simulink subsystem "rss_GDVltgHiLvl1Dia"  (R2023a)
settings: Solver=VariableStepAuto  StartTime=0.0  StopTime=10.0  RelTol=1e-3
undefined symbols (not defined in the file): ENM_TYPE_FALT, Gu16_ctGDVltgHiLvl1ConfCnt_C, Gu16_ctGDVltgHiLvl1RcvyCnt_C, Gu16_uGDVltgHiLvl1ConfTrs_C, Gu16_uGDVltgHiLvl1RcvyTrs_C
libraries: vhit_control_library x1, lib_debounce x1, lib_fault_definiteness x1
settings Model: Creator=xiaoqiang.yuan  LastModifiedBy=xiaoqiang.yuan

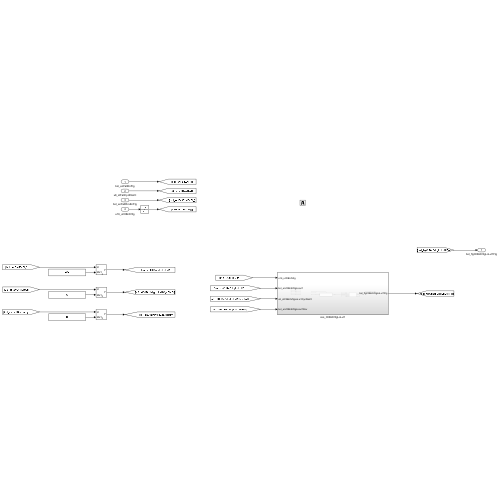
[thumbnail: Simulink's stored preview of the top-level diagram]
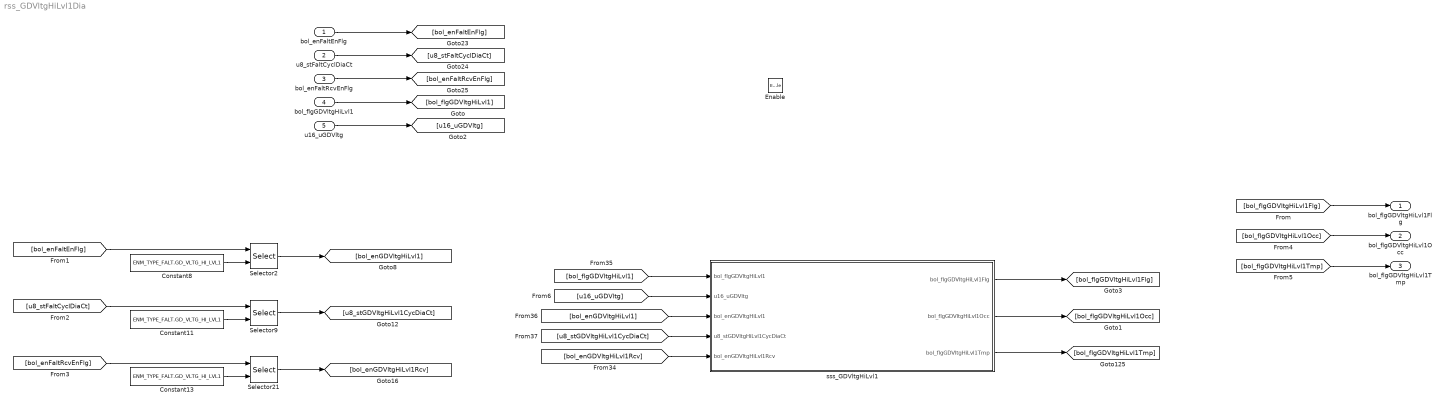
== system rss_GDVltgHiLvl1Dia ==
  bol_enFaltEnFlg : Inport  OutDataTypeStr=boolean
  u8_stFaltCyclDiaCt : Inport  Port=2  OutDataTypeStr=uint8
  bol_enFaltRcvEnFlg : Inport  Port=3  OutDataTypeStr=boolean
  bol_flgGDVltgHiLvl1 : Inport  Port=4  OutDataTypeStr=boolean
  u16_uGDVltg : Inport  Port=5  OutDataTypeStr=dt_Standardize_u16p15b0
  Enable : EnablePort
  Constant11 : Constant  Value=ENM_TYPE_FALT.GD_VLTG_HI_LVL1
  Constant13 : Constant  Value=ENM_TYPE_FALT.GD_VLTG_HI_LVL1
  Constant8 : Constant  Value=ENM_TYPE_FALT.GD_VLTG_HI_LVL1
  Selector2 : Selector  IndexMode=Zero-based  InputPortWidth=Cdbl_numFaltDiaNum  IndexOptions=Index vector (port)  Indices=[1 3]  OutputSizes=1
  Selector21 : Selector  IndexMode=Zero-based  InputPortWidth=Cdbl_numFaltDiaNum  IndexOptions=Index vector (port)  Indices=[1 3]  OutputSizes=1
  Selector9 : Selector  IndexMode=Zero-based  InputPortWidth=Cdbl_numFaltDiaNum  IndexOptions=Index vector (port)  Indices=[1 3]  OutputSizes=1
  sss_GDVltgHiLvl1 : Subsystem
  bol_flgGDVltgHiLvl1Flg : Outport  OutDataTypeStr=boolean
  bol_flgGDVltgHiLvl1Occ : Outport  Port=2  OutDataTypeStr=boolean
  bol_flgGDVltgHiLvl1Tmp : Outport  Port=3  OutDataTypeStr=boolean
  wires:
  [bol_flgGDVltgHiLvl1Flg] -> bol_flgGDVltgHiLvl1Flg/1
  [bol_flgGDVltgHiLvl1] -> sss_GDVltgHiLvl1/1(bol_flgGDVltgHiLvl1)
  [u8_stGDVltgHiLvl1CycDiaCt] -> sss_GDVltgHiLvl1/4(u8_stGDVltgHiLvl1CycDiaCt)
  [bol_enGDVltgHiLvl1] -> sss_GDVltgHiLvl1/3(bol_enGDVltgHiLvl1)
  sss_GDVltgHiLvl1/1(bol_flgGDVltgHiLvl1Flg) -> [bol_flgGDVltgHiLvl1Flg]
  [bol_enGDVltgHiLvl1Rcv] -> sss_GDVltgHiLvl1/5(bol_enGDVltgHiLvl1Rcv)
  u8_stFaltCyclDiaCt/1 -> [u8_stFaltCyclDiaCt]
  bol_enFaltRcvEnFlg/1 -> [bol_enFaltRcvEnFlg]
  bol_enFaltEnFlg/1 -> [bol_enFaltEnFlg]
  [u8_stFaltCyclDiaCt] -> Selector9/1
  [bol_enFaltRcvEnFlg] -> Selector21/1
  [bol_enFaltEnFlg] -> Selector2/1
  Selector21/1 -> [bol_enGDVltgHiLvl1Rcv]
  Selector9/1 -> [u8_stGDVltgHiLvl1CycDiaCt]
  Selector2/1 -> [bol_enGDVltgHiLvl1]
  Constant11/1 -> Selector9/2
  Constant13/1 -> Selector21/2
  Constant8/1 -> Selector2/2
  bol_flgGDVltgHiLvl1/1 -> [bol_flgGDVltgHiLvl1]
  sss_GDVltgHiLvl1/2(bol_flgGDVltgHiLvl1Occ) -> [bol_flgGDVltgHiLvl1Occ]
  [bol_flgGDVltgHiLvl1Occ] -> bol_flgGDVltgHiLvl1Occ/1
  [u16_uGDVltg] -> sss_GDVltgHiLvl1/2(u16_uGDVltg)
  u16_uGDVltg/1 -> [u16_uGDVltg]
  [bol_flgGDVltgHiLvl1Tmp] -> bol_flgGDVltgHiLvl1Tmp/1
  sss_GDVltgHiLvl1/3(bol_flgGDVltgHiLvl1Tmp) -> [bol_flgGDVltgHiLvl1Tmp]

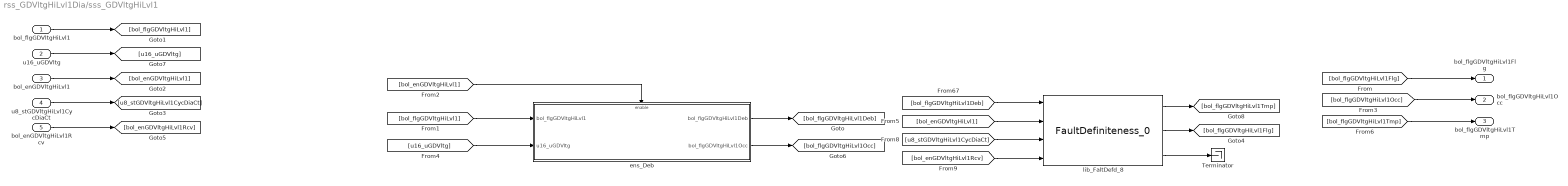
== system rss_GDVltgHiLvl1Dia/sss_GDVltgHiLvl1 ==
  bol_flgGDVltgHiLvl1 : Inport
  u16_uGDVltg : Inport  Port=2
  bol_enGDVltgHiLvl1 : Inport  Port=3
  u8_stGDVltgHiLvl1CycDiaCt : Inport  Port=4
  bol_enGDVltgHiLvl1Rcv : Inport  Port=5
  Terminator : Terminator
  ens_Deb : Subsystem  Variant=on  VariantControlMode=label  VariantControl=Choice  LabelModeActiveChoice=GEELY_PROJECT
  lib_FaltDefd_8 : lib_fault_definiteness/FaultDefiniteness_0  lb_FaltWaitRecvCnt=Gu16_ctGDVltgHiLvl1ConfCnt_C
  bol_flgGDVltgHiLvl1Flg : Outport
  bol_flgGDVltgHiLvl1Occ : Outport  Port=2
  bol_flgGDVltgHiLvl1Tmp : Outport  Port=3
  wires:
  [bol_flgGDVltgHiLvl1Tmp] -> bol_flgGDVltgHiLvl1Tmp/1
  [u16_uGDVltg] -> ens_Deb/2(u16_uGDVltg)
  u16_uGDVltg/1 -> [u16_uGDVltg]
  ens_Deb/2(bol_flgGDVltgHiLvl1Occ) -> [bol_flgGDVltgHiLvl1Occ]
  ens_Deb/1(bol_flgGDVltgHiLvl1Deb) -> [bol_flgGDVltgHiLvl1Deb]
  [bol_enGDVltgHiLvl1] -> ens_Deb/Enable
  [bol_flgGDVltgHiLvl1] -> ens_Deb/1(bol_flgGDVltgHiLvl1)
  [bol_flgGDVltgHiLvl1Occ] -> bol_flgGDVltgHiLvl1Occ/1
  lib_FaltDefd_8/1 -> [bol_flgGDVltgHiLvl1Tmp]
  lib_FaltDefd_8/2 -> [bol_flgGDVltgHiLvl1Flg]
  lib_FaltDefd_8/3 -> Terminator/1
  bol_enGDVltgHiLvl1Rcv/1 -> [bol_enGDVltgHiLvl1Rcv]
  u8_stGDVltgHiLvl1CycDiaCt/1 -> [u8_stGDVltgHiLvl1CycDiaCt]
  bol_enGDVltgHiLvl1/1 -> [bol_enGDVltgHiLvl1]
  [bol_flgGDVltgHiLvl1Flg] -> bol_flgGDVltgHiLvl1Flg/1
  bol_flgGDVltgHiLvl1/1 -> [bol_flgGDVltgHiLvl1]
  [bol_enGDVltgHiLvl1Rcv] -> lib_FaltDefd_8/4
  [u8_stGDVltgHiLvl1CycDiaCt] -> lib_FaltDefd_8/3
  [bol_enGDVltgHiLvl1] -> lib_FaltDefd_8/2
  [bol_flgGDVltgHiLvl1Deb] -> lib_FaltDefd_8/1

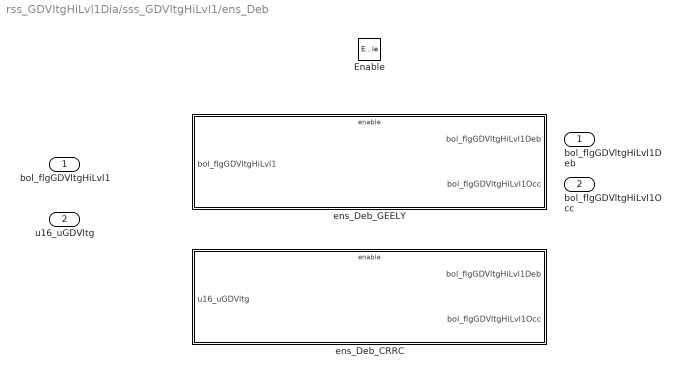
== system rss_GDVltgHiLvl1Dia/sss_GDVltgHiLvl1/ens_Deb ==
  bol_flgGDVltgHiLvl1 : Inport
  u16_uGDVltg : Inport  Port=2
  Enable : EnablePort
  ens_Deb_CRRC : Subsystem  VariantControl=CRRC_PROJECT
  ens_Deb_GEELY : Subsystem  VariantControl=GEELY_PROJECT
  bol_flgGDVltgHiLvl1Deb : Outport
  bol_flgGDVltgHiLvl1Occ : Outport  Port=2

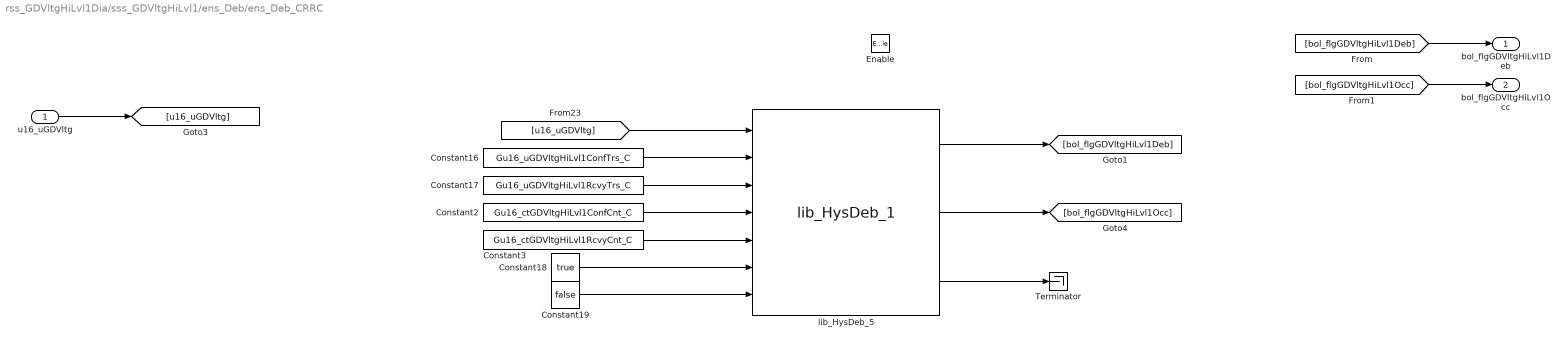
== system rss_GDVltgHiLvl1Dia/sss_GDVltgHiLvl1/ens_Deb/ens_Deb_CRRC ==
  u16_uGDVltg : Inport
  Enable : EnablePort
  Constant16 : Constant  Value=Gu16_uGDVltgHiLvl1ConfTrs_C
  Constant17 : Constant  Value=Gu16_uGDVltgHiLvl1RcvyTrs_C
  Constant18 : Constant  Value=true  OutDataTypeStr=boolean
  Constant19 : Constant  Value=false  OutDataTypeStr=boolean
  Constant2 : Constant  Value=Gu16_ctGDVltgHiLvl1ConfCnt_C
  Constant3 : Constant  Value=Gu16_ctGDVltgHiLvl1RcvyCnt_C
  Terminator : Terminator
  lib_HysDeb_5 : vhit_control_library/lib_HysDeb_1  lb_parInitOutp=0
  bol_flgGDVltgHiLvl1Deb : Outport
  bol_flgGDVltgHiLvl1Occ : Outport  Port=2
  wires:
  lib_HysDeb_5/1 -> [bol_flgGDVltgHiLvl1Deb]
  [u16_uGDVltg] -> lib_HysDeb_5/1
  Constant17/1 -> lib_HysDeb_5/3
  Constant18/1 -> lib_HysDeb_5/6
  lib_HysDeb_5/3 -> Terminator/1
  Constant2/1 -> lib_HysDeb_5/4
  Constant19/1 -> lib_HysDeb_5/7
  Constant16/1 -> lib_HysDeb_5/2
  Constant3/1 -> lib_HysDeb_5/5
  lib_HysDeb_5/2 -> [bol_flgGDVltgHiLvl1Occ]
  [bol_flgGDVltgHiLvl1Deb] -> bol_flgGDVltgHiLvl1Deb/1
  [bol_flgGDVltgHiLvl1Occ] -> bol_flgGDVltgHiLvl1Occ/1
  u16_uGDVltg/1 -> [u16_uGDVltg]

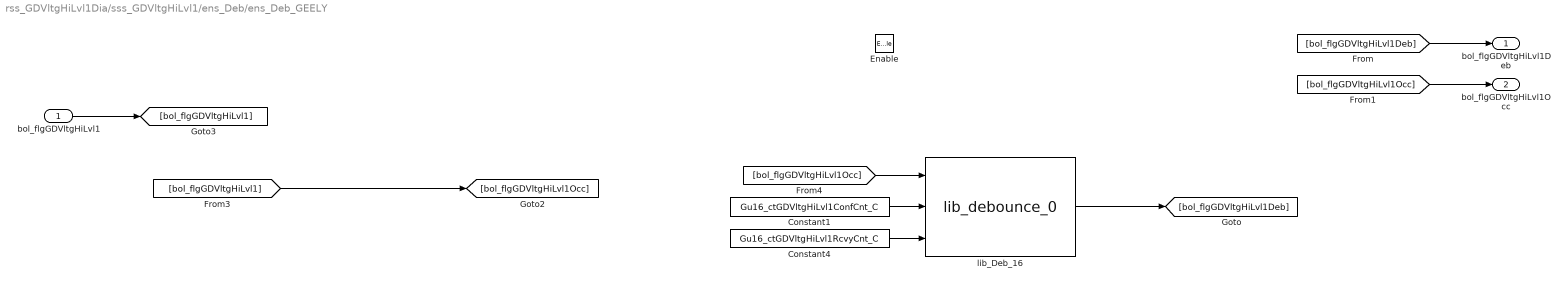
== system rss_GDVltgHiLvl1Dia/sss_GDVltgHiLvl1/ens_Deb/ens_Deb_GEELY ==
  bol_flgGDVltgHiLvl1 : Inport
  Enable : EnablePort
  Constant1 : Constant  Value=Gu16_ctGDVltgHiLvl1ConfCnt_C
  Constant4 : Constant  Value=Gu16_ctGDVltgHiLvl1RcvyCnt_C
  lib_Deb_16 : lib_debounce/lib_debounce_0
  bol_flgGDVltgHiLvl1Deb : Outport
  bol_flgGDVltgHiLvl1Occ : Outport  Port=2
  wires:
  bol_flgGDVltgHiLvl1/1 -> [bol_flgGDVltgHiLvl1]
  [bol_flgGDVltgHiLvl1Occ] -> lib_Deb_16/1
  lib_Deb_16/1 -> [bol_flgGDVltgHiLvl1Deb]
  Constant1/1 -> lib_Deb_16/2
  Constant4/1 -> lib_Deb_16/3
  [bol_flgGDVltgHiLvl1] -> [bol_flgGDVltgHiLvl1Occ]
  [bol_flgGDVltgHiLvl1Occ] -> bol_flgGDVltgHiLvl1Occ/1
  [bol_flgGDVltgHiLvl1Deb] -> bol_flgGDVltgHiLvl1Deb/1
